simulink model "AMC_BLDC"  (R2023b)
settings: configuration reference "AMCBLDC_Configuration" (kept outside this file)
settings Model: DataDictionary=amcbldc.sldd  VariantConfigurationObject=MCVariants  Creator=upattacini  LastModifiedBy=mfussi
settings ConfigSetRef: SourceName=AMCBLDC_Configuration

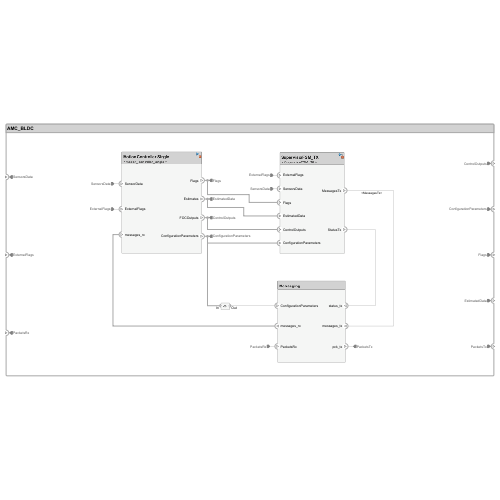
[thumbnail: Simulink's stored preview of the top-level diagram]
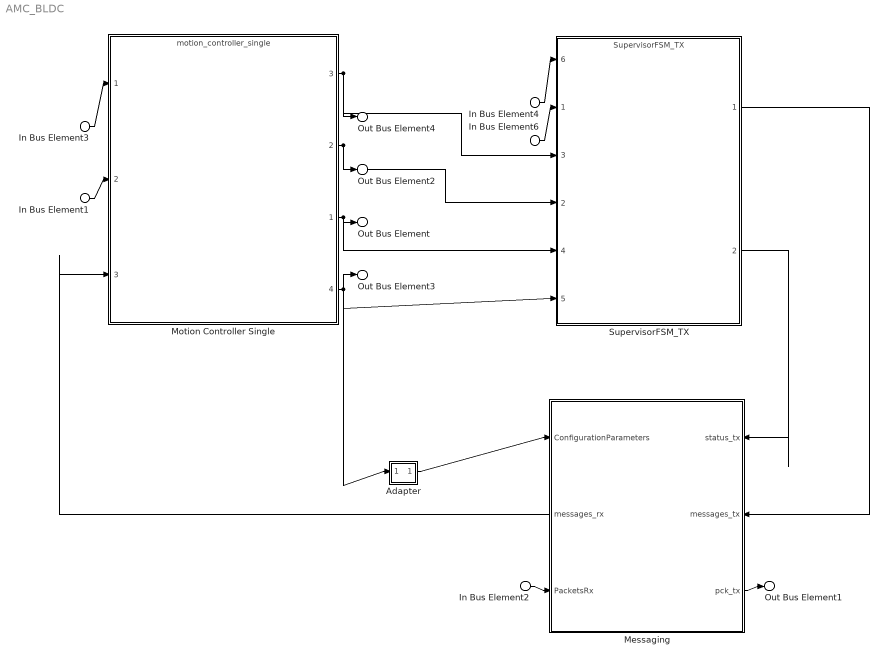
== system AMC_BLDC ==
  In Bus Element6 : Inport  PortName=SensorsData
  In Bus Element3 : Inport  PortName=SensorsData
  In Bus Element4 : Inport  Port=2  PortName=ExternalFlags
  In Bus Element1 : Inport  Port=2  PortName=ExternalFlags
  In Bus Element2 : Inport  Port=3  PortName=PacketsRx
  Adapter : Subsystem
      settings: PortSchema="{\"entries\":[{\"content\":{\"margin\":10,\"minimumSpacing\":15,\"sides\":[{\"content\":{\"connectorIds\":[\"In1\"]},\"type\":\"ConnectorPlacement.EquallySpacedRectSide\",\"uuid\":\"86e9389d-5838-4074-8501-a63cbbaf12b3\"},{\"content\":{\"connectorIds\":[\"Out1\"],\"side\":\"RIGHT\"},\"type\":\"ConnectorPlacement.EquallySpacedRectSide\",\"uuid\":\"f002dbfd-8113-450a-8d26-ec1606cc6892\"},{\"content\":{\"side\":\"TOP\"},\"type\":\"ConnectorPlacement.EquallySpacedRectSide\",\"uuid\":\"ac2b1175-2c79-4a9d-8ee3-9ed07d7777c4\"}]},\"type\":\"ConnectorPlacement.EquallySpacedConnector\",\"uuid\":\"34eadedd-3176-45eb-87d3-6ff8896d8548\"}],\"packageUris\":[\"http://schema.mathworks.com/mf0/Connector/R2020b\"],\"version\":\"1.0\"}"
  Messaging : Subsystem
      settings: PortSchema="{\"entries\":[{\"content\":{\"headerSize\":26,\"margin\":15,\"minimumSpacing\":25,\"sides\":[{\"content\":{\"connectorIds\":[\"In3\",\"Out2\",\"In1\"]},\"type\":\"ConnectorPlacement.EquallySpacedRectSide\",\"uuid\":\"2148a9ca-a041-4019-8738-bc30807315dc\"},{\"content\":{\"connectorIds\":[\"In4\",\"In2\",\"Out1\"],\"side\":\"RIGHT\"},\"type\":\"ConnectorPlacement.EquallySpacedRectSide\",\"uuid\":\"d2884f22-8c53-43de-b638-02974377300f\"},{\"content\":{\"side\":\"TOP\"},\"type\":\"ConnectorPlacement.EquallySpacedRectSide\",\"uuid\":\"0563c894-934a-48e6-bdf6-cacba4ee5b45\"},{\"content\":{\"side\":\"BOTTOM\"},\"type\":\"ConnectorPlacement.EquallySpacedRectSide\",\"uuid\":\"9d0264c3-5ca4-4a71-92f0-4ebcad17af76\"}]},\"type\":\"ConnectorPlacement.EquallySpacedConnector\",\"uuid\":\"aceedaa9-7f20-49f1-93cc-8d7be38f8964\"}],\"packageUris\":[\"http://schema.mathworks.com/mf0/Connector/R2020b\"],\"version\":\"1.0\"}"
  Motion Controller Single : ModelReference  ModelNameDialog=motion_controller_single.slx  SimulationMode=Normal  ModelReferenceVersion=1.175
      settings: PortSchema="{\"entries\":[{\"content\":{\"headerSize\":38,\"margin\":15,\"minimumSpacing\":25,\"sides\":[{\"content\":{\"connectorIds\":[\"In1\",\"In2\",\"In3\"]},\"type\":\"ConnectorPlacement.EquallySpacedRectSide\",\"uuid\":\"f5cf413d-ba4f-4573-b6b7-0f383360eb97\"},{\"content\":{\"connectorIds\":[\"Out3\",\"Out2\",\"Out1\",\"Out4\"],\"side\":\"RIGHT\"},\"type\":\"ConnectorPlacement.EquallySpacedRectSide\",\"uuid\":\"fcf07879-e858-44c6-9fd7-a7efb93672a8\"},{\"content\":{\"side\":\"TOP\"},\"type\":\"ConnectorPlacement.EquallySpacedRectSide\",\"uuid\":\"51210f80-623a-465a-bb18-6978a9da34ce\"},{\"content\":{\"side\":\"BOTTOM\"},\"type\":\"ConnectorPlacement.EquallySpacedRectSide\",\"uuid\":\"f15bf243-0eb7-466e-91ce-b70aec3f50bc\"}]},\"type\":\"ConnectorPlacement.EquallySpacedConnector\",\"uuid\":\"25ffebdb-746b-4ae0-8cae-cea39d2d3aef\"}],\"packageUris\":[\"http://schema.mathworks.com/mf0/Connector/R2020b\"],\"version\":\"1.0\"}"
  SupervisorFSM_TX : ModelReference  ModelNameDialog=SupervisorFSM_TX.slx  SimulationMode=Normal  ModelReferenceVersion=7.17
      settings: PortSchema="{\"entries\":[{\"content\":{\"headerSize\":38,\"margin\":15,\"minimumSpacing\":25,\"sides\":[{\"content\":{\"connectorIds\":[\"In6\",\"In1\",\"In3\",\"In2\",\"In4\",\"In5\"]},\"type\":\"ConnectorPlacement.EquallySpacedRectSide\",\"uuid\":\"4aedf767-9c1b-4c88-bc72-7777321bcd41\"},{\"content\":{\"connectorIds\":[\"Out1\",\"Out2\"],\"side\":\"RIGHT\"},\"type\":\"ConnectorPlacement.EquallySpacedRectSide\",\"uuid\":\"aee88cc0-e097-47ae-97af-9ad4a0a9b7bf\"},{\"content\":{\"side\":\"TOP\"},\"type\":\"ConnectorPlacement.EquallySpacedRectSide\",\"uuid\":\"173fabf3-9ac1-4c2f-9d1c-2c077518d79f\"},{\"content\":{\"side\":\"HIDDEN\"},\"type\":\"ConnectorPlacement.EquallySpacedRectSide\",\"uuid\":\"c63b284f-1c4e-4f1a-bde6-4ce5f749d319\"}]},\"type\":\"ConnectorPlacement.EquallySpacedConnector\",\"uuid\":\"40fdf982-cc0d-4196-8efc-330d112bcb29\"}],\"packageUris\":[\"http://schema.mathworks.com/mf0/Connector/R2020b\"],\"version\":\"1.0\"}"
  Out Bus Element : Outport  PortName=ControlOutputs
  Out Bus Element3 : Outport  Port=2  PortName=ConfigurationParameters
  Out Bus Element4 : Outport  Port=3  PortName=Flags
  Out Bus Element2 : Outport  Port=4  PortName=EstimatedData
  Out Bus Element1 : Outport  Port=5  PortName=PacketsTx
  wires:
  In Bus Element2/1 -> Messaging/1(PacketsRx)
  Messaging/1(pck_tx) -> Out Bus Element1/1
  Motion Controller Single/4 -> SupervisorFSM_TX/5, Out Bus Element3/1, Adapter/1(In)
  SupervisorFSM_TX/2 -> Messaging/4(status_tx)
  SupervisorFSM_TX/1 -> Messaging/2(messages_tx)
  In Bus Element6/1 -> SupervisorFSM_TX/1
  Motion Controller Single/1 -> Out Bus Element/1, SupervisorFSM_TX/4
  Motion Controller Single/2 -> Out Bus Element2/1, SupervisorFSM_TX/2
  Motion Controller Single/3 -> Out Bus Element4/1, SupervisorFSM_TX/3
  In Bus Element3/1 -> Motion Controller Single/1
  In Bus Element4/1 -> SupervisorFSM_TX/6
  Adapter/1(Out) -> Messaging/3(ConfigurationParameters)
  In Bus Element1/1 -> Motion Controller Single/2
  Messaging/2(messages_rx) -> Motion Controller Single/3

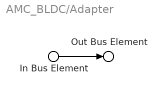
== system AMC_BLDC/Adapter ==
  In Bus Element : Inport  PortName=In
  Out Bus Element : Outport  PortName=Out
  wires:
  In Bus Element/1 -> Out Bus Element/1

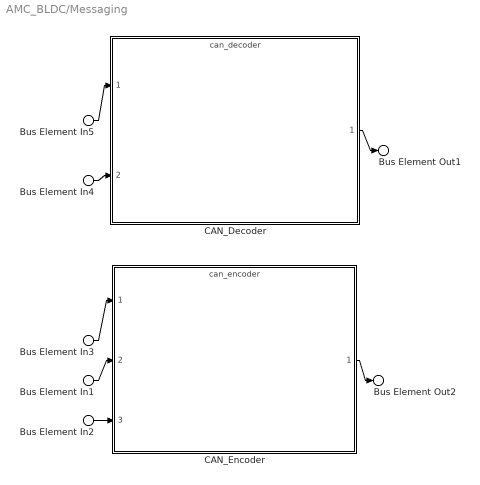
== system AMC_BLDC/Messaging ==
  Bus Element In5 : Inport  PortName=PacketsRx
  Bus Element In3 : Inport  Port=2  PortName=messages_tx
  Bus Element In2 : Inport  Port=3  PortName=ConfigurationParameters
  Bus Element In4 : Inport  Port=3  PortName=ConfigurationParameters
  Bus Element In1 : Inport  Port=4  PortName=status_tx
  CAN_Decoder : ModelReference  ModelNameDialog=can_decoder  SimulationMode=Normal  ModelReferenceVersion=6.115
      settings: PortSchema="{\"entries\":[{\"content\":{\"headerSize\":38,\"margin\":15,\"minimumSpacing\":25,\"sides\":[{\"content\":{\"connectorIds\":[\"In1\",\"In2\"]},\"type\":\"ConnectorPlacement.EquallySpacedRectSide\",\"uuid\":\"b2b94824-c700-4373-91d8-47add34cc094\"},{\"content\":{\"connectorIds\":[\"Out1\"],\"side\":\"RIGHT\"},\"type\":\"ConnectorPlacement.EquallySpacedRectSide\",\"uuid\":\"93c2845f-b99b-4543-8e08-c46ac526332e\"},{\"content\":{\"side\":\"TOP\"},\"type\":\"ConnectorPlacement.EquallySpacedRectSide\",\"uuid\":\"58bbde8c-049b-4e4b-9306-530fa2daad17\"}]},\"type\":\"ConnectorPlacement.EquallySpacedConnector\",\"uuid\":\"2d51588d-c4d7-43f4-87c2-9173ed7811d6\"}],\"packageUris\":[\"http://schema.mathworks.com/mf0/Connector/R2020b\"],\"version\":\"1.0\"}"
  CAN_Encoder : ModelReference  ModelNameDialog=can_encoder  SimulationMode=Normal  ModelReferenceVersion=6.9
      settings: PortSchema="{\"entries\":[{\"content\":{\"headerSize\":38,\"margin\":15,\"minimumSpacing\":25,\"sides\":[{\"content\":{\"connectorIds\":[\"In1\",\"In2\",\"In3\"]},\"type\":\"ConnectorPlacement.EquallySpacedRectSide\",\"uuid\":\"6f4b08cd-f6c5-49bf-b1cb-2cd7d6623be6\"},{\"content\":{\"connectorIds\":[\"Out1\"],\"side\":\"RIGHT\"},\"type\":\"ConnectorPlacement.EquallySpacedRectSide\",\"uuid\":\"50a4d36e-deb5-40a6-b950-d37a57b313ee\"},{\"content\":{\"connectorIds\":[],\"side\":\"TOP\"},\"type\":\"ConnectorPlacement.EquallySpacedRectSide\",\"uuid\":\"f26608a5-c459-46f7-8e1f-f1e374dcdcf6\"}]},\"type\":\"ConnectorPlacement.EquallySpacedConnector\",\"uuid\":\"e591c604-78a1-48e3-93c5-357c40d96f0b\"}],\"packageUris\":[\"http://schema.mathworks.com/mf0/Connector/R2020b\"],\"version\":\"1.0\"}"
  Bus Element Out2 : Outport  PortName=pck_tx
  Bus Element Out1 : Outport  Port=2  PortName=messages_rx
  wires:
  Bus Element In3/1 -> CAN_Encoder/1
  Bus Element In1/1 -> CAN_Encoder/2
  CAN_Encoder/1 -> Bus Element Out2/1
  Bus Element In5/1 -> CAN_Decoder/1
  Bus Element In2/1 -> CAN_Encoder/3
  Bus Element In4/1 -> CAN_Decoder/2
  CAN_Decoder/1 -> Bus Element Out1/1
